simulink model "AV_7_zadacha2_NATRUPUVANJE_NA_INTEGRALNA_KOMPONENTA"  (R2018a)
settings: Solver=VariableStepAuto  StartTime=0.0  StopTime=1500  RelTol=1e-3
libraries: simulink_extras x2
settings Model: Creator=DD  LastModifiedBy=DD

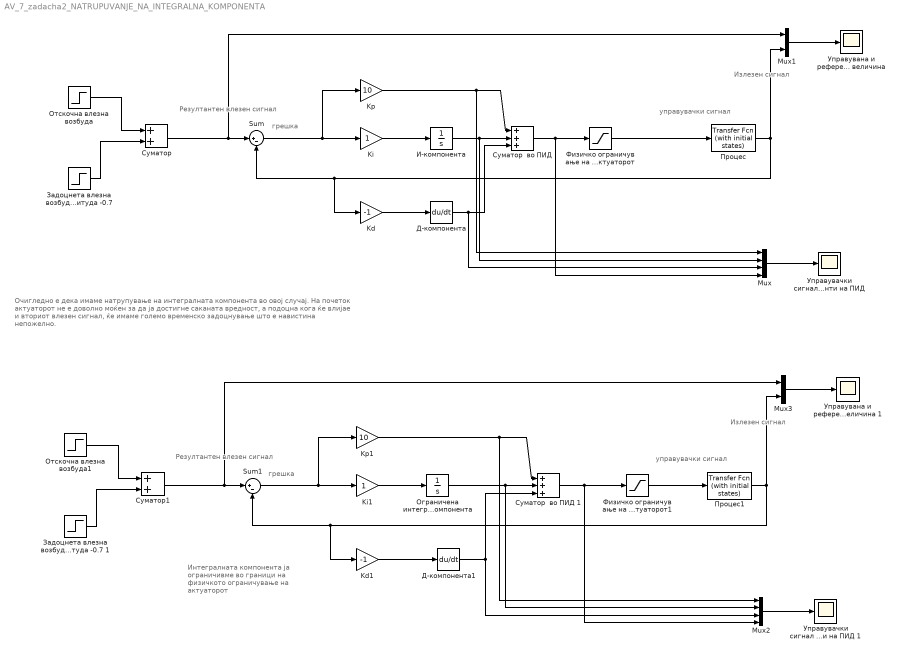
== system AV_7_zadacha2_NATRUPUVANJE_NA_INTEGRALNA_KOMPONENTA ==
  note: Интегралната компонента ја ограничивме во граници на физичкото ограничување на актуаторот
  note: Очигледно е дека имаме натрупување на интегралната компонента во овој случај.
      | На почеток актуаторот не е доволно моќен за да ја достигне саканата вредност, а подоцна
      | кога ќе влијае и вториот влезен сигнал, ќе имаме големо временско задоцнување што е навистина непожелно.
  note: Излезен
      | сигнал
  note: управувачки сигнал
  note: грешка
  note: Резултантен влезен сигнал
  note: Резултантен влезен сигнал
  note: управувачки сигнал
  note: грешка
  note: Излезен
      | сигнал
  " Процес" : simulink_extras/Additional Linear/Transfer Fcn (with initial states)  N=[1]  D="[1  10 20]"  X0=.5
  " Процес1" : simulink_extras/Additional Linear/Transfer Fcn (with initial states)  N=[1]  D="[1  10 20]"  X0=.5
  Kd : Gain  Gain=-1
  Kd1 : Gain  Gain=-1
  Ki : Gain
  Ki1 : Gain
  Kp : Gain  Gain=10
  Kp1 : Gain  Gain=10
  Mux : Mux
  Mux1 : Mux  Inputs=2
  Mux2 : Mux
  Mux3 : Mux  Inputs=2
  Sum : Sum  Inputs=|+-
  Sum1 : Sum  Inputs=|+-
  Д-компонента : Derivative
  Д-компонента1 : Derivative
  "Задоцнета влезна возбуда со амплитуда -0.7 " : Step  Time=300  After=-0.7  SampleTime=0
  Задоцнета влезна возбуда со амплитуда -0.7 1 : Step  Time=300  After=-0.7  SampleTime=0
  И-компонента : Integrator
  Ограничена интегрална компонента : Integrator  LimitOutput=on  UpperSaturationLimit=10  LowerSaturationLimit=-10
  Отскочна влезна возбуда : Step  SampleTime=0
  Отскочна влезна возбуда1 : Step  SampleTime=0
  Суматор : Sum
  "Суматор  во ПИД " : Sum  Inputs=+++
  Суматор  во ПИД 1 : Sum  Inputs=+++
  Суматор1 : Sum
  "Управувана и референтна величина " : Scope
  Управувана и референтна величина 1 : Scope
  "Управувачки сигнал Поединечни компоненти на ПИД " : Scope
  Управувачки сигнал Поединечни компоненти на ПИД 1 : Scope
  Физичко ограничување на актуаторот : Saturate  UpperLimit=10  LowerLimit=-10
  Физичко ограничување на актуаторот1 : Saturate  UpperLimit=10  LowerLimit=-10
  wires:
  "Задоцнета влезна возбуда со амплитуда -0.7 "/1 -> Суматор/2
  Отскочна влезна возбуда/1 -> Суматор/1
  Суматор/1 -> Mux1/1, Sum/1
  Sum/1 -> Kp/1, Ki/1
  Kd/1 -> Д-компонента/1
  Ki/1 -> И-компонента/1
  И-компонента/1 -> Mux/2, "Суматор  во ПИД "/2
  Kp/1 -> Mux/1, "Суматор  во ПИД "/1
  Д-компонента/1 -> Mux/3, "Суматор  во ПИД "/3
  "Суматор  во ПИД "/1 -> Mux/4, Физичко ограничување на актуаторот/1
  " Процес"/1 -> Mux1/2, Kd/1, Sum/2
  Mux1/1 -> "Управувана и референтна величина "/1
  Mux/1 -> "Управувачки сигнал Поединечни компоненти на ПИД "/1
  Физичко ограничување на актуаторот/1 -> " Процес"/1
  Отскочна влезна возбуда1/1 -> Суматор1/1
  Ограничена интегрална компонента/1 -> Mux2/2, Суматор  во ПИД 1/2
  Kp1/1 -> Mux2/1, Суматор  во ПИД 1/1
  Суматор  во ПИД 1/1 -> Mux2/4, Физичко ограничување на актуаторот1/1
  Задоцнета влезна возбуда со амплитуда -0.7 1/1 -> Суматор1/2
  Kd1/1 -> Д-компонента1/1
  Суматор1/1 -> Mux3/1, Sum1/1
  Sum1/1 -> Kp1/1, Ki1/1
  " Процес1"/1 -> Mux3/2, Kd1/1, Sum1/2
  Mux3/1 -> Управувана и референтна величина 1/1
  Д-компонента1/1 -> Mux2/3, Суматор  во ПИД 1/3
  Ki1/1 -> Ограничена интегрална компонента/1
  Физичко ограничување на актуаторот1/1 -> " Процес1"/1
  Mux2/1 -> Управувачки сигнал Поединечни компоненти на ПИД 1/1
